simulink model "Testmodell"  (R2017b)
settings: Solver=ode45  StartTime=0.0  StopTime=1220  RelTol=1e-3  EnableMultiTasking=on
undefined symbols (not defined in the file): eta_EM_map, T_EM_max, w_EM_row, w_EM_upper
libraries: simulink x4, qss_tb_library x3
settings Model: Creator=donya  LastModifiedBy=Flugk
settings DataIOCC: LimitDataPoints=on  SaveFormat=Array
settings OptimizationCC: LifeSpan=inf
settings DebuggingCC: SolverPrmCheckMsg=warning  SFUnexpectedBacktrackingDiag=warning  SFNoUnconditionalDefaultTransitionDiag=warning  SFExecutionAtInitializationDiag=none
settings HardwareCC: ProdBitPerPointer=32  ProdBitPerSizeT=32  ProdBitPerPtrDiffT=32  ProdLargestAtomicFloat=None  ProdIntDivRoundTo=Undefined  ProdEndianess=Unspecified  ProdWordSize=32  ProdHWDeviceType=32-bit Generic
settings ModelReferenceCC: PropagateSignalLabelsOutOfModel=off
settings CodeAppCC: StateflowObjectComments=on
settings GRTTargetCC: TargetLangStandard=C89/C90 (ANSI)  GeneratePreprocessorConditionals=Disable all
settings ConfigComp: CovMetricSettings=dw  CovHtmlReporting=on  CovSaveCumulativeToWorkspaceVar=on  CovSaveSingleToWorkspaceVar=on  CovExternalEMLEnable=off  CovSFcnEnable=off

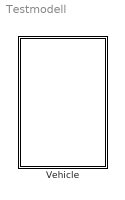
== system Testmodell ==
  Vehicle : Subsystem

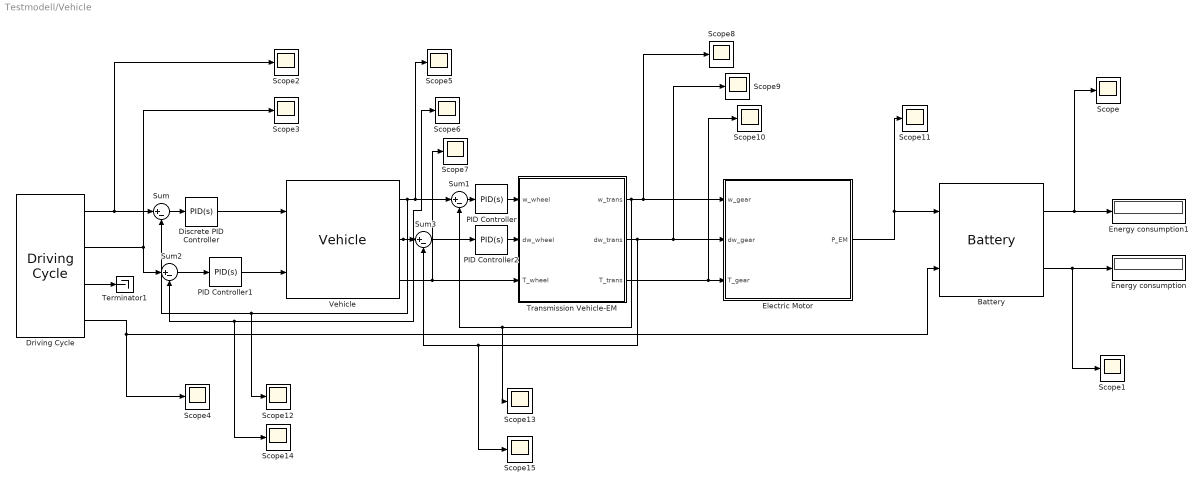
== system Testmodell/Vehicle ==
  Battery : qss_tb_library/Energy Buffer/Battery  Tag=battery  I_0=100  Q_BT_IC_rel=27.78  t_ch=20
  Discrete PID Controller : simulink/Continuous/PID Controller  Controller=PID  TimeDomain=Continuous-time  SampleTime=-1  IntegratorMethod=Forward Euler  FilterMethod=Forward Euler  Form=Parallel  UseFilter=on  ControllerParametersSource=internal  P=1  I=1  D=0  N=100  InitialConditionSource=internal  InitialConditionForIntegrator=0  InitialConditionForFilter=0  ExternalReset=none  LimitOutput=off  UpperSaturationLimit=inf  LowerSaturationLimit=-inf  LinearizeAsGain=off  AntiWindupMode=none  Kb=1  TrackingMode=off  Kt=1  PParamMin=[]  PParamMax=[]  IParamMin=[]  IParamMax=[]  DParamMin=[]  DParamMax=[]  NParamMin=[]  NParamMax=[]  KbParamMin=[]  KbParamMax=[]  KtParamMin=[]  KtParamMax=[]  POutMin=[]  POutMax=[]  IOutMin=[]  IOutMax=[]  DOutMin=[]  DOutMax=[]  NOutMin=[]  NOutMax=[]  KbOutMin=[]  KbOutMax=[]  KtOutMin=[]  KtOutMax=[]  IntegratorOutMin=[]  IntegratorOutMax=[]  FilterOutMin=[]  FilterOutMax=[]  SumOutMin=[]  SumOutMax=[]  SumI1OutMin=[]  SumI1OutMax=[]  SumI2OutMin=[]  SumI2OutMax=[]  SumI3OutMin=[]  SumI3OutMax=[]  SumDOutMin=[]  SumDOutMax=[]  SaturationOutMin=[]  SaturationOutMax=[]  IntegratorContinuousStateAttributes=''  IntegratorStateMustResolveToSignalObject=off  IntegratorRTWStateStorageClass=Auto  FilterContinuousStateAttributes=''  FilterStateMustResolveToSignalObject=off  FilterRTWStateStorageClass=Auto  DifferentiatorICPrevScaledInput=0  DifferentiatorOutMin=[]  DifferentiatorOutMax=[]  InitialConditionSetting=State (most efficient)  FilterDiffOutCoefMin=[]  FilterDiffOutCoefMax=[]  SumDenOutMin=[]  SumDenOutMax=[]  SumNumOutMin=[]  SumNumOutMax=[]  ReciprocalOutMin=[]  ReciprocalOutMax=[]  DivideOutMin=[]  DivideOutMax=[]  TunerSelectOption=Transfer Function Based (PID Tuner App)
  Driving Cycle : qss_tb_library/Driving Cycle/Driving Cycle  Tag=cycle  cyclenr=Europe: NEDC  stepsize=1  autostop=on
  Electric Motor : Subsystem  AncestorBlock=qss_tb_library/Energy Converter/Electric Motor  mask(Electric Motor){scale_EM=3.5, theta_EM=0.1, P_aux=0}
      mask prompts: scale_EM "Motor scaling factor [-]"; theta_EM "Motor inertia [kg*m2]"; P_aux "Power required by auxiliaries [W]"
      mask help:
      | This block simulates the behaviour of an electric motor. The block is based on an efficiency map.
      |
      | Input:
      | =====
      | 	w_gear		Speed of the fly wheel [rad/s]
      | 	dw_gear	Acceleration of the fly wheel [rad/s^2]
      | 	T_gear		Torque on the fly wheel [Nm]
      |
      | Output:
      | ======
      | 	P_EM		Power produced by the electric motor [W]
      mask init:
      | init_EM;
  Energy consumption : Display
  Energy consumption1 : Display
  PID Controller : simulink/Continuous/PID Controller  Controller=PID  TimeDomain=Continuous-time  SampleTime=-1  IntegratorMethod=Forward Euler  FilterMethod=Forward Euler  Form=Parallel  UseFilter=on  ControllerParametersSource=internal  P=1  I=1  D=0  N=100  InitialConditionSource=internal  InitialConditionForIntegrator=0  InitialConditionForFilter=0  ExternalReset=none  LimitOutput=off  UpperSaturationLimit=inf  LowerSaturationLimit=-inf  LinearizeAsGain=on  AntiWindupMode=none  Kb=1  TrackingMode=off  Kt=1  PParamMin=[]  PParamMax=[]  IParamMin=[]  IParamMax=[]  DParamMin=[]  DParamMax=[]  NParamMin=[]  NParamMax=[]  KbParamMin=[]  KbParamMax=[]  KtParamMin=[]  KtParamMax=[]  POutMin=[]  POutMax=[]  IOutMin=[]  IOutMax=[]  DOutMin=[]  DOutMax=[]  NOutMin=[]  NOutMax=[]  KbOutMin=[]  KbOutMax=[]  KtOutMin=[]  KtOutMax=[]  IntegratorOutMin=[]  IntegratorOutMax=[]  FilterOutMin=[]  FilterOutMax=[]  SumOutMin=[]  SumOutMax=[]  SumI1OutMin=[]  SumI1OutMax=[]  SumI2OutMin=[]  SumI2OutMax=[]  SumI3OutMin=[]  SumI3OutMax=[]  SumDOutMin=[]  SumDOutMax=[]  SaturationOutMin=[]  SaturationOutMax=[]  IntegratorContinuousStateAttributes=''  IntegratorStateMustResolveToSignalObject=off  IntegratorRTWStateStorageClass=Auto  FilterContinuousStateAttributes=''  FilterStateMustResolveToSignalObject=off  FilterRTWStateStorageClass=Auto  DifferentiatorICPrevScaledInput=0  DifferentiatorOutMin=[]  DifferentiatorOutMax=[]  InitialConditionSetting=State (most efficient)  FilterDiffOutCoefMin=[]  FilterDiffOutCoefMax=[]  SumDenOutMin=[]  SumDenOutMax=[]  SumNumOutMin=[]  SumNumOutMax=[]  ReciprocalOutMin=[]  ReciprocalOutMax=[]  DivideOutMin=[]  DivideOutMax=[]  TunerSelectOption=Transfer Function Based (PID Tuner App)
  PID Controller1 : simulink/Continuous/PID Controller  Controller=PID  TimeDomain=Continuous-time  SampleTime=-1  IntegratorMethod=Forward Euler  FilterMethod=Forward Euler  Form=Parallel  UseFilter=on  ControllerParametersSource=internal  P=1  I=1  D=0  N=100  InitialConditionSource=internal  InitialConditionForIntegrator=0  InitialConditionForFilter=0  ExternalReset=none  LimitOutput=off  UpperSaturationLimit=inf  LowerSaturationLimit=-inf  LinearizeAsGain=on  AntiWindupMode=none  Kb=1  TrackingMode=off  Kt=1  PParamMin=[]  PParamMax=[]  IParamMin=[]  IParamMax=[]  DParamMin=[]  DParamMax=[]  NParamMin=[]  NParamMax=[]  KbParamMin=[]  KbParamMax=[]  KtParamMin=[]  KtParamMax=[]  POutMin=[]  POutMax=[]  IOutMin=[]  IOutMax=[]  DOutMin=[]  DOutMax=[]  NOutMin=[]  NOutMax=[]  KbOutMin=[]  KbOutMax=[]  KtOutMin=[]  KtOutMax=[]  IntegratorOutMin=[]  IntegratorOutMax=[]  FilterOutMin=[]  FilterOutMax=[]  SumOutMin=[]  SumOutMax=[]  SumI1OutMin=[]  SumI1OutMax=[]  SumI2OutMin=[]  SumI2OutMax=[]  SumI3OutMin=[]  SumI3OutMax=[]  SumDOutMin=[]  SumDOutMax=[]  SaturationOutMin=[]  SaturationOutMax=[]  IntegratorContinuousStateAttributes=''  IntegratorStateMustResolveToSignalObject=off  IntegratorRTWStateStorageClass=Auto  FilterContinuousStateAttributes=''  FilterStateMustResolveToSignalObject=off  FilterRTWStateStorageClass=Auto  DifferentiatorICPrevScaledInput=0  DifferentiatorOutMin=[]  DifferentiatorOutMax=[]  InitialConditionSetting=State (most efficient)  FilterDiffOutCoefMin=[]  FilterDiffOutCoefMax=[]  SumDenOutMin=[]  SumDenOutMax=[]  SumNumOutMin=[]  SumNumOutMax=[]  ReciprocalOutMin=[]  ReciprocalOutMax=[]  DivideOutMin=[]  DivideOutMax=[]  TunerSelectOption=Transfer Function Based (PID Tuner App)
  PID Controller2 : simulink/Continuous/PID Controller  Controller=PID  TimeDomain=Continuous-time  SampleTime=-1  IntegratorMethod=Forward Euler  FilterMethod=Forward Euler  Form=Parallel  UseFilter=on  ControllerParametersSource=internal  P=1  I=1  D=0  N=100  InitialConditionSource=internal  InitialConditionForIntegrator=0  InitialConditionForFilter=0  ExternalReset=none  LimitOutput=off  UpperSaturationLimit=inf  LowerSaturationLimit=-inf  LinearizeAsGain=on  AntiWindupMode=none  Kb=1  TrackingMode=off  Kt=1  PParamMin=[]  PParamMax=[]  IParamMin=[]  IParamMax=[]  DParamMin=[]  DParamMax=[]  NParamMin=[]  NParamMax=[]  KbParamMin=[]  KbParamMax=[]  KtParamMin=[]  KtParamMax=[]  POutMin=[]  POutMax=[]  IOutMin=[]  IOutMax=[]  DOutMin=[]  DOutMax=[]  NOutMin=[]  NOutMax=[]  KbOutMin=[]  KbOutMax=[]  KtOutMin=[]  KtOutMax=[]  IntegratorOutMin=[]  IntegratorOutMax=[]  FilterOutMin=[]  FilterOutMax=[]  SumOutMin=[]  SumOutMax=[]  SumI1OutMin=[]  SumI1OutMax=[]  SumI2OutMin=[]  SumI2OutMax=[]  SumI3OutMin=[]  SumI3OutMax=[]  SumDOutMin=[]  SumDOutMax=[]  SaturationOutMin=[]  SaturationOutMax=[]  IntegratorContinuousStateAttributes=''  IntegratorStateMustResolveToSignalObject=off  IntegratorRTWStateStorageClass=Auto  FilterContinuousStateAttributes=''  FilterStateMustResolveToSignalObject=off  FilterRTWStateStorageClass=Auto  DifferentiatorICPrevScaledInput=0  DifferentiatorOutMin=[]  DifferentiatorOutMax=[]  InitialConditionSetting=State (most efficient)  FilterDiffOutCoefMin=[]  FilterDiffOutCoefMax=[]  SumDenOutMin=[]  SumDenOutMax=[]  SumNumOutMin=[]  SumNumOutMax=[]  ReciprocalOutMin=[]  ReciprocalOutMax=[]  DivideOutMin=[]  DivideOutMax=[]  TunerSelectOption=Transfer Function Based (PID Tuner App)
  Scope{,1..15} (16 alike) : Scope
  Sum{,1..3} (4 alike) : Sum  Inputs=|+-
  Terminator1 : Terminator
  Transmission Vehicle-EM : Subsystem  Tag=simple transmission  AncestorBlock=qss_tb_library/Gear System/Transmission  mask(Transmission){gear_ratio=3.5, e_GT=0.98, P_GT0=300, w_wheel_min=1}
      mask prompts: gear_ratio "Gear ratio [-]"; e_GT "Efficiency [-]"; P_GT0 "Idling losses (friction) [W]"; w_wheel_min "Minimum wheel speed beyond which losses are generated [rad/s]"
      mask help:
      | This block simulates a transmission with a fixed gear ratio.
      |
      | Input:
      | =====
      | 	w_wheel	Speed of the wheel [rad/s]
      | 	dw_wheel	Acceleration of the wheel [rad/s^2]
      | 	T_wheel	Torque on the wheel [Nm]
      |
      | Output:
      | ======
      | 	w_trans		Speed of the fly wheel [rad/s]
      | 	dw_trans	Acceleration of the fly wheel [rad/s^2]
      | 	T_trans		Torque on the fly wheel [Nm]
      mask init:
      | init_transmission;
  Vehicle : qss_tb_library/Vehicle/Vehicle  Tag=vehicle  m_f=474  mt2m_f=5  A_f=1.59  d_wheel=0.265  cw=0.26  mu=0.008
  wires:
  Transmission Vehicle-EM/1(w_trans) -> Scope13/1, Sum1/2, Scope8/1, Electric Motor/1(w_gear)
  Driving Cycle/3 -> Terminator1/1
  Electric Motor/1(P_EM) -> Scope11/1, Battery/1
  Driving Cycle/4 -> Scope4/1, Battery/2
  Battery/2 -> Scope1/1, Energy consumption/1
  Driving Cycle/2 -> Sum2/1, Scope3/1
  Battery/1 -> Scope/1, Energy consumption1/1
  Vehicle/1 -> Sum1/1, Scope5/1, Scope12/1, Sum/2
  Discrete PID Controller/1 -> Vehicle/1
  Driving Cycle/1 -> Sum/1, Scope2/1
  Sum/1 -> Discrete PID Controller/1
  PID Controller/1 -> Transmission Vehicle-EM/1(w_wheel)
  Sum1/1 -> PID Controller/1
  Sum2/1 -> PID Controller1/1
  PID Controller1/1 -> Vehicle/2
  Vehicle/2 -> Scope14/1, Sum2/2, Scope6/1, Sum3/1
  Sum3/1 -> PID Controller2/1
  PID Controller2/1 -> Transmission Vehicle-EM/2(dw_wheel)
  Transmission Vehicle-EM/2(dw_trans) -> Scope15/1, Sum3/2, Scope9/1, Electric Motor/2(dw_gear)
  Vehicle/3 -> Transmission Vehicle-EM/3(T_wheel), Scope7/1
  Transmission Vehicle-EM/3(T_trans) -> Scope10/1, Electric Motor/3(T_gear)

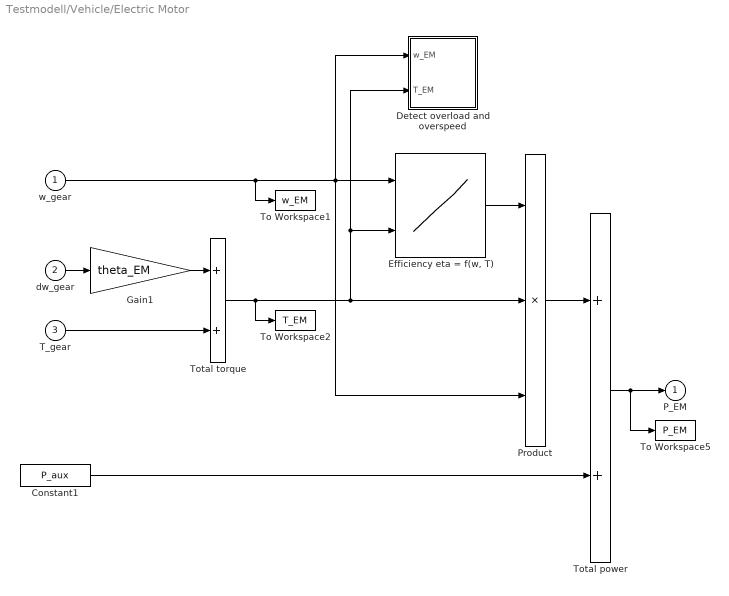
== system Testmodell/Vehicle/Electric Motor ==
  w_gear : Inport
  dw_gear : Inport  Port=2
  T_gear : Inport  Port=3
  Constant1 : Constant  Value=P_aux
  Detect overload and overspeed : Subsystem
  "Efficiency eta = f(w, T)" : Lookup2D  RowIndex=w_EM_row  ColumnIndex=T_EM_col  Table=eta_EM_map
  Gain1 : Gain  Gain=theta_EM  SaturateOnIntegerOverflow=on  OutDataTypeStr=Inherit: Same as input  ParamDataTypeStr=Inherit: Same as input
  Product : Product  Inputs=3  SaturateOnIntegerOverflow=on  RndMeth=Zero  InputSameDT=on  OutDataTypeStr=Inherit: Same as first input
  To Workspace1 : ToWorkspace  VariableName=w_EM  SampleTime=-1
  To Workspace2 : ToWorkspace  VariableName=T_EM  SampleTime=-1
  To Workspace5 : ToWorkspace  VariableName=P_EM  SampleTime=-1
  Total power : Sum  SaturateOnIntegerOverflow=on  InputSameDT=on  OutDataTypeStr=Inherit: Same as first input
  Total torque : Sum  SaturateOnIntegerOverflow=on  InputSameDT=on  OutDataTypeStr=Inherit: Same as first input
  P_EM : Outport  InitialOutput=0
  wires:
  Total power/1 -> To Workspace5/1, P_EM/1
  Product/1 -> Total power/1
  Constant1/1 -> Total power/2
  Total torque/1 -> To Workspace2/1, Product/2, "Efficiency eta = f(w, T)"/2, Detect overload and overspeed/2(T_EM)
  Gain1/1 -> Total torque/1
  T_gear/1 -> Total torque/2
  dw_gear/1 -> Gain1/1
  "Efficiency eta = f(w, T)"/1 -> Product/1
  w_gear/1 -> To Workspace1/1, Product/3, "Efficiency eta = f(w, T)"/1, Detect overload and overspeed/1(w_EM)

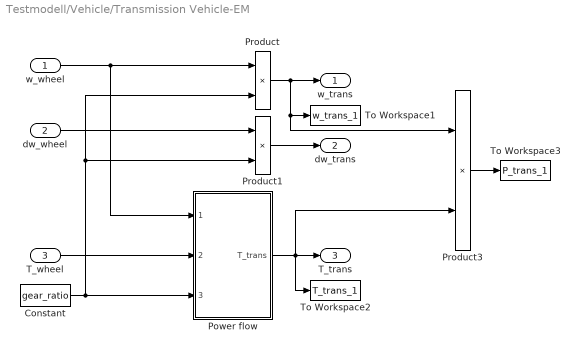
== system Testmodell/Vehicle/Transmission Vehicle-EM ==
  w_wheel : Inport
  dw_wheel : Inport  Port=2
  T_wheel : Inport  Port=3
  Constant : Constant  Value=gear_ratio
  Power flow : Subsystem
  Product : Product  SaturateOnIntegerOverflow=on  RndMeth=Zero  InputSameDT=on  OutDataTypeStr=Inherit: Same as first input
  Product1 : Product  SaturateOnIntegerOverflow=on  RndMeth=Zero  InputSameDT=on  OutDataTypeStr=Inherit: Same as first input
  Product3 : Product  SaturateOnIntegerOverflow=on  RndMeth=Zero  InputSameDT=on  OutDataTypeStr=Inherit: Same as first input
  To Workspace1 : ToWorkspace  VariableName=w_trans_1  SampleTime=-1
  To Workspace2 : ToWorkspace  VariableName=T_trans_1  SampleTime=-1
  To Workspace3 : ToWorkspace  VariableName=P_trans_1  SampleTime=-1
  w_trans : Outport  InitialOutput=0
  dw_trans : Outport  Port=2  InitialOutput=0
  T_trans : Outport  Port=3  InitialOutput=0
  wires:
  Product3/1 -> To Workspace3/1
  w_wheel/1 -> Power flow/1(w_wheel), Product/1
  Constant/1 -> Product/2, Product1/2, Power flow/3(gear_ratio)
  T_wheel/1 -> Power flow/2(T_wheel)
  dw_wheel/1 -> Product1/1
  Product/1 -> Product3/1, To Workspace1/1, w_trans/1
  Product1/1 -> dw_trans/1
  Power flow/1(T_trans) -> Product3/2, To Workspace2/1, T_trans/1

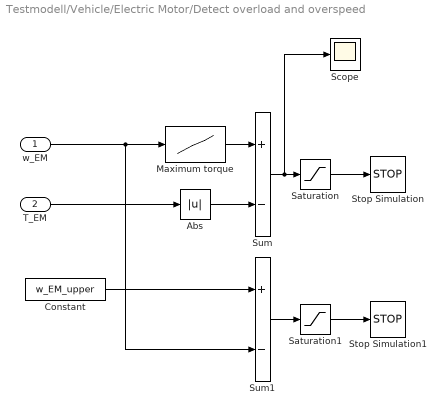
== system Testmodell/Vehicle/Electric Motor/Detect overload and overspeed ==
  w_EM : Inport
  T_EM : Inport  Port=2
  Abs : Abs  SaturateOnIntegerOverflow=on
  Constant : Constant  Value=w_EM_upper
  Maximum torque : Lookup  InputValues=w_EM_row  Table=T_EM_max  SaturateOnIntegerOverflow=on
  Saturation : Saturate  UpperLimit=0  LowerLimit=-inf
  Saturation1 : Saturate  UpperLimit=0  LowerLimit=-inf
  Scope : Scope
  Stop Simulation : Stop
  Stop Simulation1 : Stop
  Sum : Sum  Inputs=+-  SaturateOnIntegerOverflow=on  InputSameDT=on  OutDataTypeStr=Inherit: Same as first input
  Sum1 : Sum  Inputs=+-  SaturateOnIntegerOverflow=on  InputSameDT=on  OutDataTypeStr=Inherit: Same as first input
  wires:
  Sum/1 -> Scope/1, Saturation/1
  w_EM/1 -> Maximum torque/1, Sum1/2
  T_EM/1 -> Abs/1
  Maximum torque/1 -> Sum/1
  Abs/1 -> Sum/2
  Saturation/1 -> Stop Simulation/1
  Constant/1 -> Sum1/1
  Sum1/1 -> Saturation1/1
  Saturation1/1 -> Stop Simulation1/1

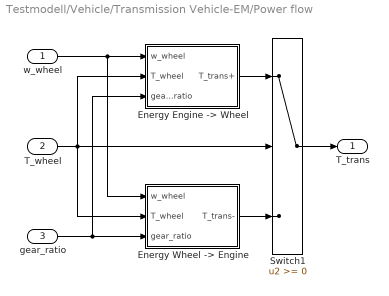
== system Testmodell/Vehicle/Transmission Vehicle-EM/Power flow ==
  w_wheel : Inport
  T_wheel : Inport  Port=2
  gear_ratio : Inport  Port=3
  "Energy Engine -> Wheel" : Subsystem
  "Energy Wheel -> Engine" : Subsystem
  Switch1 : Switch  SaturateOnIntegerOverflow=on  InputSameDT=on
  T_trans : Outport  InitialOutput=0
  wires:
  Switch1/1 -> T_trans/1
  "Energy Engine -> Wheel"/1(T_trans+) -> Switch1/1
  T_wheel/1 -> Switch1/2, "Energy Engine -> Wheel"/2(T_wheel), "Energy Wheel -> Engine"/2(T_wheel)
  "Energy Wheel -> Engine"/1(T_trans-) -> Switch1/3
  gear_ratio/1 -> "Energy Engine -> Wheel"/3(gear_ratio), "Energy Wheel -> Engine"/3(gear_ratio)
  w_wheel/1 -> "Energy Engine -> Wheel"/1(w_wheel), "Energy Wheel -> Engine"/1(w_wheel)

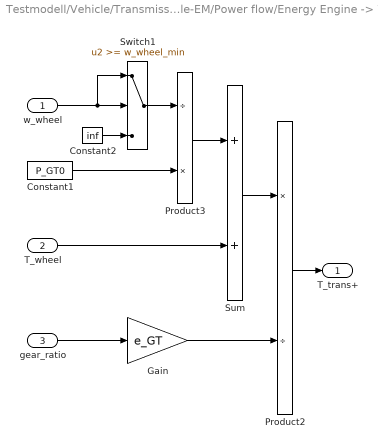
== system Testmodell/Vehicle/Transmission Vehicle-EM/Power flow/Energy Engine -> Wheel ==
  w_wheel : Inport
  T_wheel : Inport  Port=2
  gear_ratio : Inport  Port=3
  Constant1 : Constant  Value=P_GT0
  Constant2 : Constant  Value=inf
  Gain : Gain  Gain=e_GT  SaturateOnIntegerOverflow=on  OutDataTypeStr=Inherit: Same as input  ParamDataTypeStr=Inherit: Same as input
  Product2 : Product  Inputs=*/  SaturateOnIntegerOverflow=on  RndMeth=Zero  InputSameDT=on  OutDataTypeStr=Inherit: Same as first input
  Product3 : Product  Inputs=/*  SaturateOnIntegerOverflow=on  RndMeth=Zero  InputSameDT=on  OutDataTypeStr=Inherit: Same as first input
  Sum : Sum  SaturateOnIntegerOverflow=on  InputSameDT=on  OutDataTypeStr=Inherit: Same as first input
  Switch1 : Switch  Threshold=w_wheel_min  SaturateOnIntegerOverflow=on  InputSameDT=on
  T_trans+ : Outport  InitialOutput=0
  wires:
  gear_ratio/1 -> Gain/1
  Constant1/1 -> Product3/2
  Switch1/1 -> Product3/1
  Constant2/1 -> Switch1/3
  w_wheel/1 -> Switch1/1, Switch1/2
  Sum/1 -> Product2/1
  Product2/1 -> T_trans+/1
  Gain/1 -> Product2/2
  Product3/1 -> Sum/1
  T_wheel/1 -> Sum/2

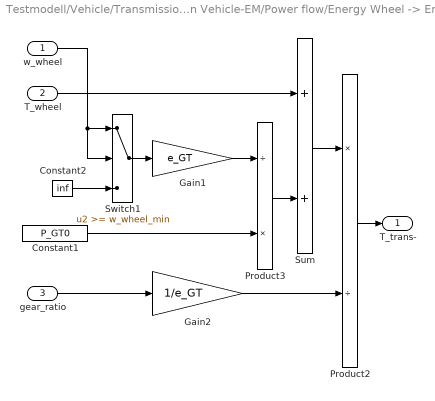
== system Testmodell/Vehicle/Transmission Vehicle-EM/Power flow/Energy Wheel -> Engine ==
  w_wheel : Inport
  T_wheel : Inport  Port=2
  gear_ratio : Inport  Port=3
  Constant1 : Constant  Value=P_GT0
  Constant2 : Constant  Value=inf
  Gain1 : Gain  Gain=e_GT  SaturateOnIntegerOverflow=on  OutDataTypeStr=Inherit: Same as input  ParamDataTypeStr=Inherit: Same as input
  Gain2 : Gain  Gain=1/e_GT  SaturateOnIntegerOverflow=on  OutDataTypeStr=Inherit: Same as input  ParamDataTypeStr=Inherit: Same as input
  Product2 : Product  Inputs=*/  SaturateOnIntegerOverflow=on  RndMeth=Zero  InputSameDT=on  OutDataTypeStr=Inherit: Same as first input
  Product3 : Product  Inputs=/*  SaturateOnIntegerOverflow=on  RndMeth=Zero  InputSameDT=on  OutDataTypeStr=Inherit: Same as first input
  Sum : Sum  SaturateOnIntegerOverflow=on  InputSameDT=on  OutDataTypeStr=Inherit: Same as first input
  Switch1 : Switch  Threshold=w_wheel_min  SaturateOnIntegerOverflow=on  InputSameDT=on
  T_trans- : Outport  InitialOutput=0
  wires:
  Gain1/1 -> Product3/1
  Sum/1 -> Product2/1
  Product3/1 -> Sum/2
  Product2/1 -> T_trans-/1
  Gain2/1 -> Product2/2
  T_wheel/1 -> Sum/1
  Constant1/1 -> Product3/2
  Switch1/1 -> Gain1/1
  Constant2/1 -> Switch1/3
  gear_ratio/1 -> Gain2/1
  w_wheel/1 -> Switch1/2, Switch1/1
